simulink model "disk_drive_intro"  (R2017a)
settings: Solver=VariableStepAuto  StartTime=0.0  StopTime=10.0  RelTol=1e-3
model workspace (MATLAB code in the model file):
  | kd = 1
  | J = 1
  | omega0 = 2
  | h = 0.4
  | a = 2*omega0
  | b = omega0/2
  | K =  2*J*omega0*omega0/kd
  | beta = K*b/a
settings Model: Creator=kjartan  LastModifiedBy=kjartan

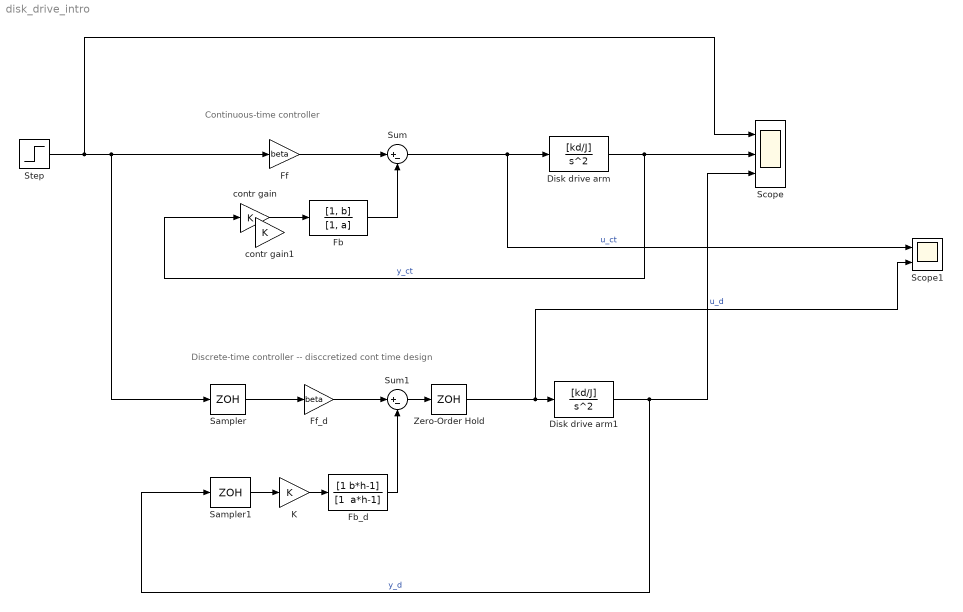
== system disk_drive_intro ==
  note: Discrete-time controller -- disccretized cont time design
  note: Continuous-time controller
  Disk drive arm : TransferFcn  Numerator=[kd/J]  Denominator=[1 0 0]
  Disk drive arm1 : TransferFcn  Numerator=[kd/J]  Denominator=[1 0 0]
  Fb : TransferFcn  Numerator=[1, b]  Denominator=[1, a]
  Fb_d : DiscreteTransferFcn  Numerator=[1 b*h-1]  Denominator="[1  a*h-1]"  SampleTime=h
  Ff : Gain  Gain=beta
  Ff_d : Gain  Gain=beta
  K : Gain  Gain=K
  Sampler : ZeroOrderHold  SampleTime=h
  Sampler1 : ZeroOrderHold  SampleTime=h
  Scope : Scope  NumInputPorts=3
  Scope1 : Scope  NumInputPorts=2
  Step : Step  Time=2*h  SampleTime=0
  Sum : Sum  Inputs=|+-
  Sum1 : Sum  Inputs=|+-
  Zero-Order Hold : ZeroOrderHold  SampleTime=h
  contr gain : Gain  Gain=K
  contr gain1 : Gain  Gain=K
  wires:
  Disk drive arm/1 -> contr gain/1, Scope/2  "y_ct"
  Sum/1 -> Scope1/1, Disk drive arm/1  "u_ct"
  Step/1 -> Ff/1, Sampler/1, Scope/1
  Disk drive arm1/1 -> Sampler1/1, Scope/3  "y_d"
  Zero-Order Hold/1 -> Scope1/2, Disk drive arm1/1  "u_d"
  Sum1/1 -> Zero-Order Hold/1
  Ff_d/1 -> Sum1/1
  Fb/1 -> Sum/2
  Ff/1 -> Sum/1
  Sampler/1 -> Ff_d/1
  Fb_d/1 -> Sum1/2
  contr gain/1 -> Fb/1
  Sampler1/1 -> K/1
  K/1 -> Fb_d/1
